simulink model "SecRwRtStHeightChk"  (R2018b)
settings: Solver=FixedStepDiscrete  StartTime=0.0  StopTime=10.0  FixedStep=0.01  RelTol=1e-3
undefined symbols (not defined in the file or in its folder): KeSMSeHeiCstTypeConfig_Val
libraries: simulink x3, HeightCalcLib x1
settings Model: Creator=sn2xws  LastModifiedBy=sn2xws
settings DataIOCC: SaveFormat=StructureWithTime
settings OptimizationCC: DefaultParameterBehavior=Inlined  EnhancedBackFolding=on  PassReuseOutputArgsAs=Individual arguments  ZeroExternalMemoryAtStartup=off  ZeroInternalMemoryAtStartup=off  OptimizeBlockOrder=speed  DifferentSizesBufferReuse=on  OptimizationCustomize=off
settings DebuggingCC: ParameterTunabilityLossMsg=error
settings ModelReferenceCC: ModelReferenceNumInstancesAllowed=Single
settings SFSimCC: MATLABDynamicMemAlloc=off
settings RTWCC: SystemTargetFile=autosar.tlc  GenCodeOnly=on  TemplateMakefile=ert_default_tmf  Description=AUTOSAR  GenerateReport=on  IncludeHyperlinkInReport=on  LaunchReport=on  GenerateTraceInfo=on  GenerateTraceReport=on  GenerateTraceReportSl=on  GenerateTraceReportSf=on  GenerateTraceReportEml=on  GenerateCodeMetricsReport=on
settings CodeAppCC: ForceParamTrailComments=on  IgnoreCustomStorageClasses=off  OperatorAnnotations=on  SimulinkDataObjDesc=on  SFDataObjDesc=on  InsertBlockDesc=on
settings STFCustomTargetCC: TargetLangStandard=C99 (ISO)  MultiwordLength=256  ParMdlRefBuildCompliant=on  CompOptLevelCompliant=on  IncludeMdlTerminateFcn=off  CombineOutputUpdateFcns=on  SuppressErrorStatus=on  ERTCustomFileBanners=on  SupportNonFinite=off  SupportComplex=off  SupportContinuousTime=off  SupportNonInlinedSFcns=off  RemoveResetFunc=on  MATLABClassNameForMDSCustomization=Simulink.SoftwareTarget.ERTCustomization  AutosarCompliant=on  UseToolchainInfoCompliant=on  LookupTableObjectStructAxisOrder=2,1,3,4,...  LUTObjectStructOrderEvenSpacing=Size,Table,Breakpoints  SystemTargetFile=autosar.tlc
settings ERTTargetCC: TargetLangStandard=C99 (ISO)  ConcurrentExecutionCompliant=off  IncludeMdlTerminateFcn=off  SuppressErrorStatus=on  SupportNonFinite=off  SupportComplex=off  ModelStepFunctionPrototypeControlCompliant=off  CPPClassGenCompliant=off  AutosarCompliant=on  LookupTableObjectStructAxisOrder=2,1,3,4,...  LUTObjectStructOrderEvenSpacing=Size,Table,Breakpoints  InlinedParameterPlacement=NonHierarchical  ERTCustomFileTemplate=example_file_process.tlc  ERTFilePackagingFormat=Compact

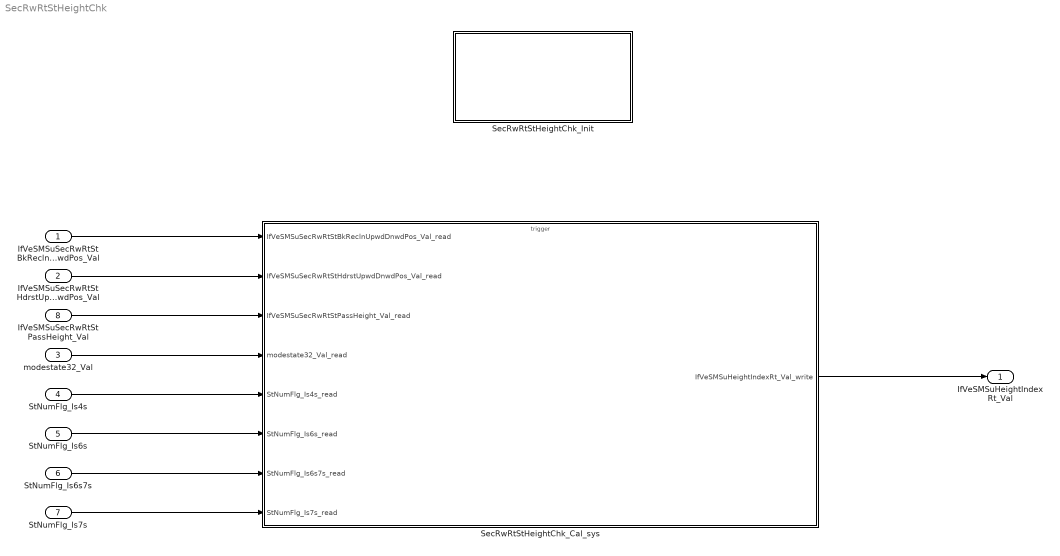
== system SecRwRtStHeightChk ==
  IfVeSMSuSecRwRtStBkReclnUpwdDnwdPos_Val : Inport  OutDataTypeStr=uint16  PortDimensions=1
  IfVeSMSuSecRwRtStHdrstUpwdDnwdPos_Val : Inport  Port=2  OutDataTypeStr=uint16  PortDimensions=1
  modestate32_Val : Inport  Port=3  OutDataTypeStr=uint32  PortDimensions=1
  StNumFlg_Is4s : Inport  Port=4  OutDataTypeStr=boolean  PortDimensions=1
  StNumFlg_Is6s : Inport  Port=5  OutDataTypeStr=boolean  PortDimensions=1
  StNumFlg_Is6s7s : Inport  Port=6  OutDataTypeStr=boolean  PortDimensions=1
  StNumFlg_Is7s : Inport  Port=7  OutDataTypeStr=boolean  PortDimensions=1
  IfVeSMSuSecRwRtStPassHeight_Val : Inport  Port=8  OutDataTypeStr=uint8  PortDimensions=1
  SecRwRtStHeightChk_Cal_sys : Subsystem
  SecRwRtStHeightChk_Init : Subsystem
  IfVeSMSuHeightIndexRt_Val : Outport  Description=|  OutDataTypeStr=uint8  PortDimensions=1
      | 0：under 160
      | 1：160
      | 2：165
      | 3：170
      | 4：175
      | 5：180
      | 6：over 180
  wires:
  IfVeSMSuSecRwRtStBkReclnUpwdDnwdPos_Val/1 -> SecRwRtStHeightChk_Cal_sys/1(IfVeSMSuSecRwRtStBkReclnUpwdDnwdPos_Val_read)
  IfVeSMSuSecRwRtStHdrstUpwdDnwdPos_Val/1 -> SecRwRtStHeightChk_Cal_sys/2(IfVeSMSuSecRwRtStHdrstUpwdDnwdPos_Val_read)
  modestate32_Val/1 -> SecRwRtStHeightChk_Cal_sys/4(modestate32_Val_read)
  StNumFlg_Is4s/1 -> SecRwRtStHeightChk_Cal_sys/5(StNumFlg_Is4s_read)
  StNumFlg_Is6s/1 -> SecRwRtStHeightChk_Cal_sys/6(StNumFlg_Is6s_read)
  StNumFlg_Is6s7s/1 -> SecRwRtStHeightChk_Cal_sys/7(StNumFlg_Is6s7s_read)
  StNumFlg_Is7s/1 -> SecRwRtStHeightChk_Cal_sys/8(StNumFlg_Is7s_read)
  IfVeSMSuSecRwRtStPassHeight_Val/1 -> SecRwRtStHeightChk_Cal_sys/3(IfVeSMSuSecRwRtStPassHeight_Val_read)
  SecRwRtStHeightChk_Cal_sys/1(IfVeSMSuHeightIndexRt_Val_write) -> IfVeSMSuHeightIndexRt_Val/1

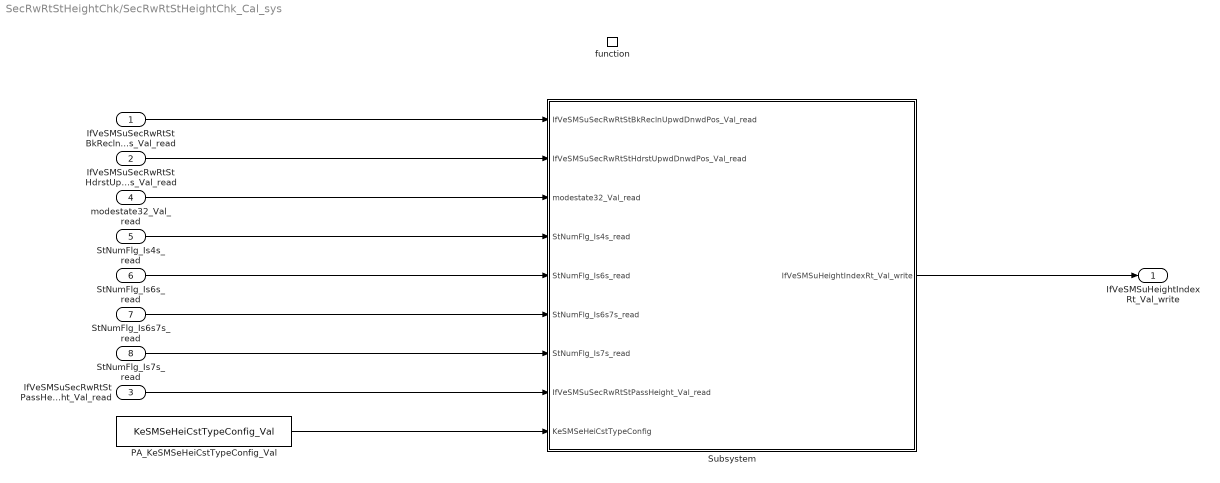
== system SecRwRtStHeightChk/SecRwRtStHeightChk_Cal_sys ==
  IfVeSMSuSecRwRtStBkReclnUpwdDnwdPos_Val_read : Inport
  IfVeSMSuSecRwRtStHdrstUpwdDnwdPos_Val_read : Inport  Port=2
  IfVeSMSuSecRwRtStPassHeight_Val_read : Inport  Port=3
  modestate32_Val_read : Inport  Port=4
  StNumFlg_Is4s_read : Inport  Port=5
  StNumFlg_Is6s_read : Inport  Port=6
  StNumFlg_Is6s7s_read : Inport  Port=7
  StNumFlg_Is7s_read : Inport  Port=8
  function : TriggerPort  TriggerType=function-call  IsSimulinkFunction=on  FunctionName=SecRwRtStHeightChk_Cal  VariantControl=(inherit)
  PA_KeSMSeHeiCstTypeConfig_Val : Constant  Value=KeSMSeHeiCstTypeConfig_Val
  Subsystem : Subsystem
  IfVeSMSuHeightIndexRt_Val_write : Outport
      settings: EnsureOutportIsVirtual=on
  wires:
  PA_KeSMSeHeiCstTypeConfig_Val/1 -> Subsystem/9(KeSMSeHeiCstTypeConfig)
  Subsystem/1(IfVeSMSuHeightIndexRt_Val_write) -> IfVeSMSuHeightIndexRt_Val_write/1
  IfVeSMSuSecRwRtStBkReclnUpwdDnwdPos_Val_read/1 -> Subsystem/1(IfVeSMSuSecRwRtStBkReclnUpwdDnwdPos_Val_read)
  IfVeSMSuSecRwRtStHdrstUpwdDnwdPos_Val_read/1 -> Subsystem/2(IfVeSMSuSecRwRtStHdrstUpwdDnwdPos_Val_read)
  modestate32_Val_read/1 -> Subsystem/3(modestate32_Val_read)
  StNumFlg_Is4s_read/1 -> Subsystem/4(StNumFlg_Is4s_read)
  StNumFlg_Is6s_read/1 -> Subsystem/5(StNumFlg_Is6s_read)
  StNumFlg_Is6s7s_read/1 -> Subsystem/6(StNumFlg_Is6s7s_read)
  StNumFlg_Is7s_read/1 -> Subsystem/7(StNumFlg_Is7s_read)
  IfVeSMSuSecRwRtStPassHeight_Val_read/1 -> Subsystem/8(IfVeSMSuSecRwRtStPassHeight_Val_read)

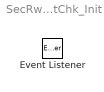
== system SecRwRtStHeightChk/SecRwRtStHeightChk_Init ==
  Event Listener : EventListener  EventName=reset

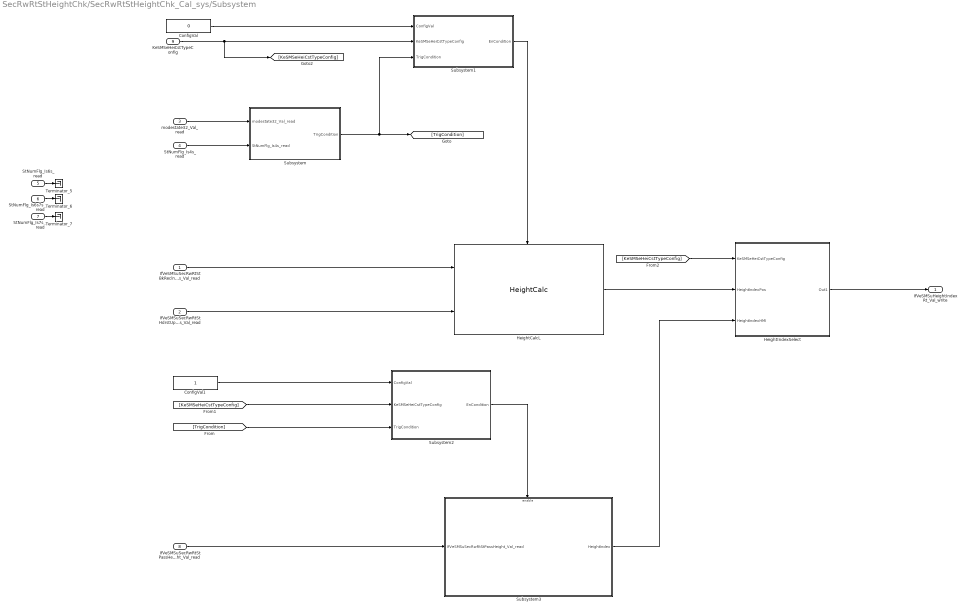
== system SecRwRtStHeightChk/SecRwRtStHeightChk_Cal_sys/Subsystem ==
  IfVeSMSuSecRwRtStBkReclnUpwdDnwdPos_Val_read : Inport
  IfVeSMSuSecRwRtStHdrstUpwdDnwdPos_Val_read : Inport  Port=2
  modestate32_Val_read : Inport  Port=3
  StNumFlg_Is4s_read : Inport  Port=4
  StNumFlg_Is6s_read : Inport  Port=5
  StNumFlg_Is6s7s_read : Inport  Port=6
  StNumFlg_Is7s_read : Inport  Port=7
  IfVeSMSuSecRwRtStPassHeight_Val_read : Inport  Port=8
  KeSMSeHeiCstTypeConfig : Inport  Port=9
  ConfigVal : Constant  Value=0  OutDataTypeStr=uint8
  ConfigVal1 : Constant  OutDataTypeStr=uint8
  HeightCalcL : HeightCalcLib/HeightCalc  SystemSampleTime=-1
  HeightIndexSelect : Subsystem
  Subsystem : Subsystem
  Subsystem1 : Subsystem
  Subsystem2 : Subsystem
  Subsystem3 : Subsystem
  Terminator_5 : Terminator
  Terminator_6 : Terminator
  Terminator_7 : Terminator
  IfVeSMSuHeightIndexRt_Val_write : Outport
      settings: EnsureOutportIsVirtual=on
  wires:
  IfVeSMSuSecRwRtStBkReclnUpwdDnwdPos_Val_read/1 -> HeightCalcL/1
  IfVeSMSuSecRwRtStHdrstUpwdDnwdPos_Val_read/1 -> HeightCalcL/2
  StNumFlg_Is6s_read/1 -> Terminator_5/1
  StNumFlg_Is7s_read/1 -> Terminator_7/1
  StNumFlg_Is6s7s_read/1 -> Terminator_6/1
  modestate32_Val_read/1 -> Subsystem/1(modestate32_Val_read)
  StNumFlg_Is4s_read/1 -> Subsystem/2(StNumFlg_Is4s_read)
  Subsystem1/1(EnCondition) -> HeightCalcL/Enable
  ConfigVal/1 -> Subsystem1/1(ConfigVal)
  ConfigVal1/1 -> Subsystem2/1(ConfigVal)
  KeSMSeHeiCstTypeConfig/1 -> [KeSMSeHeiCstTypeConfig], Subsystem1/2(KeSMSeHeiCstTypeConfig)
  [TrigCondition] -> Subsystem2/3(TrigCondition)
  [KeSMSeHeiCstTypeConfig] -> Subsystem2/2(KeSMSeHeiCstTypeConfig)
  IfVeSMSuSecRwRtStPassHeight_Val_read/1 -> Subsystem3/1(IfVeSMSuSecRwRtStPassHeight_Val_read)
  Subsystem2/1(EnCondition) -> Subsystem3/Enable
  HeightCalcL/1 -> HeightIndexSelect/2(HeightIndexPos)
  Subsystem3/1(HeightIndex) -> HeightIndexSelect/3(HeightIndexHMI)
  HeightIndexSelect/1(Out1) -> IfVeSMSuHeightIndexRt_Val_write/1
  [KeSMSeHeiCstTypeConfig] -> HeightIndexSelect/1(KeSMSeHeiCstTypeConfig)
  Subsystem/1(TrigCondition) -> [TrigCondition], Subsystem1/3(TrigCondition)

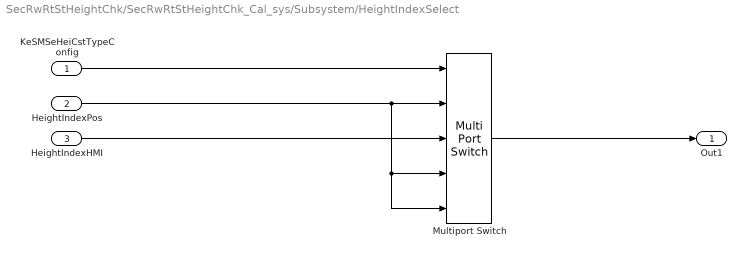
== system SecRwRtStHeightChk/SecRwRtStHeightChk_Cal_sys/Subsystem/HeightIndexSelect ==
  KeSMSeHeiCstTypeConfig : Inport
  HeightIndexPos : Inport  Port=2
  HeightIndexHMI : Inport  Port=3
  Multiport Switch : MultiPortSwitch  DataPortOrder=Zero-based contiguous  DataPortForDefault=Additional data port  DiagnosticForDefault=None  zeroidx=on
  Out1 : Outport
  wires:
  HeightIndexPos/1 -> Multiport Switch/5, Multiport Switch/4, Multiport Switch/2
  KeSMSeHeiCstTypeConfig/1 -> Multiport Switch/1
  Multiport Switch/1 -> Out1/1
  HeightIndexHMI/1 -> Multiport Switch/3

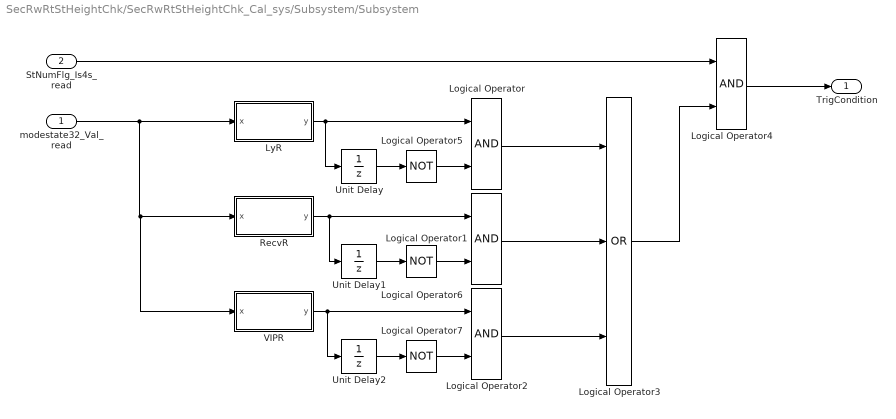
== system SecRwRtStHeightChk/SecRwRtStHeightChk_Cal_sys/Subsystem/Subsystem ==
  modestate32_Val_read : Inport
  StNumFlg_Is4s_read : Inport  Port=2
  Logical Operator{,1..2,4} (4 alike) : Logic  AllPortsSameDT=off  OutDataTypeStr=boolean
  Logical Operator3 : Logic  Operator=OR  Inputs=3  AllPortsSameDT=off  OutDataTypeStr=boolean
  Logical Operator5 : Logic  Operator=NOT  AllPortsSameDT=off  OutDataTypeStr=boolean
  Logical Operator6 : Logic  Operator=NOT  AllPortsSameDT=off  OutDataTypeStr=boolean
  Logical Operator7 : Logic  Operator=NOT  AllPortsSameDT=off  OutDataTypeStr=boolean
  LyR : Subsystem  mask(32 Bit Selector){BitNum=14}
      mask prompts: BitNum "Select Bit Number"
      mask help: Allows selection of a particular bit (0-31) out of a packed word up to 32 bits long. Output will be true if the bit number selected via the mask parameter is equal to one.
      mask TypeOptions BitNum: 0 | 1 | 2 | 3 | 4 | 5 | 6 | 7 | 8 | 9 | 10 | 11 | 12 | 13 | 14 | 15 | 16 | 17 | 18 | 19 | 20 | 21 | 22 | 23 | 24 | 25 | 26 | 27 | 28 | 29 | 30 | 31
      mask Display:
      | text(0.5, 0.8,'BIT','horizontalAlignment','center')
      | text(0.5, 0.5,'SELECTOR','horizontalAlignment','center')
      | text(0.5, 0.2,['-- Bit ',char(get_param(gcb,'BitNum')),' --'],'horizontalAlignment','center')
  RecvR : Subsystem  mask(32 Bit Selector){BitNum=12}
      mask prompts: BitNum "Select Bit Number"
      mask help: Allows selection of a particular bit (0-31) out of a packed word up to 32 bits long. Output will be true if the bit number selected via the mask parameter is equal to one.
      mask TypeOptions BitNum: 0 | 1 | 2 | 3 | 4 | 5 | 6 | 7 | 8 | 9 | 10 | 11 | 12 | 13 | 14 | 15 | 16 | 17 | 18 | 19 | 20 | 21 | 22 | 23 | 24 | 25 | 26 | 27 | 28 | 29 | 30 | 31
      mask Display:
      | text(0.5, 0.8,'BIT','horizontalAlignment','center')
      | text(0.5, 0.5,'SELECTOR','horizontalAlignment','center')
      | text(0.5, 0.2,['-- Bit ',char(get_param(gcb,'BitNum')),' --'],'horizontalAlignment','center')
  Unit Delay : UnitDelay  SampleTime=-1
  Unit Delay1 : UnitDelay  SampleTime=-1
  Unit Delay2 : UnitDelay  SampleTime=-1
  VIPR : Subsystem  mask(32 Bit Selector){BitNum=11}
      mask prompts: BitNum "Select Bit Number"
      mask help: Allows selection of a particular bit (0-31) out of a packed word up to 32 bits long. Output will be true if the bit number selected via the mask parameter is equal to one.
      mask TypeOptions BitNum: 0 | 1 | 2 | 3 | 4 | 5 | 6 | 7 | 8 | 9 | 10 | 11 | 12 | 13 | 14 | 15 | 16 | 17 | 18 | 19 | 20 | 21 | 22 | 23 | 24 | 25 | 26 | 27 | 28 | 29 | 30 | 31
      mask Display:
      | text(0.5, 0.8,'BIT','horizontalAlignment','center')
      | text(0.5, 0.5,'SELECTOR','horizontalAlignment','center')
      | text(0.5, 0.2,['-- Bit ',char(get_param(gcb,'BitNum')),' --'],'horizontalAlignment','center')
  TrigCondition : Outport
  wires:
  VIPR/1(y) -> Unit Delay2/1, Logical Operator2/1
  RecvR/1(y) -> Unit Delay1/1, Logical Operator1/1
  StNumFlg_Is4s_read/1 -> Logical Operator4/1
  LyR/1(y) -> Unit Delay/1, Logical Operator/1
  Logical Operator2/1 -> Logical Operator3/3
  modestate32_Val_read/1 -> VIPR/1(x), RecvR/1(x), LyR/1(x)
  Logical Operator3/1 -> Logical Operator4/2
  Logical Operator1/1 -> Logical Operator3/2
  Logical Operator/1 -> Logical Operator3/1
  Logical Operator4/1 -> TrigCondition/1
  Unit Delay/1 -> Logical Operator5/1
  Logical Operator5/1 -> Logical Operator/2
  Unit Delay1/1 -> Logical Operator6/1
  Logical Operator6/1 -> Logical Operator1/2
  Unit Delay2/1 -> Logical Operator7/1
  Logical Operator7/1 -> Logical Operator2/2

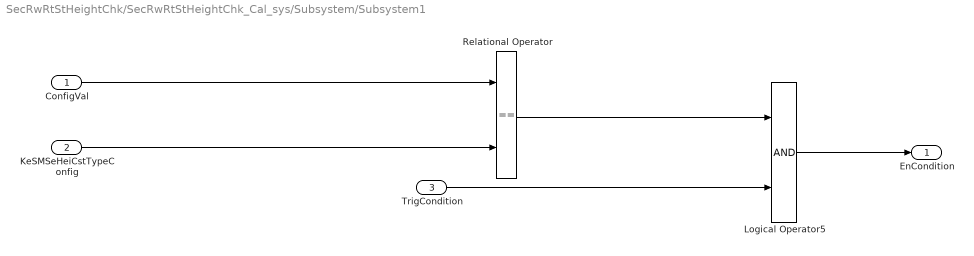
== system SecRwRtStHeightChk/SecRwRtStHeightChk_Cal_sys/Subsystem/Subsystem1 ==
  ConfigVal : Inport
  KeSMSeHeiCstTypeConfig : Inport  Port=2
  TrigCondition : Inport  Port=3
  Logical Operator5 : Logic  AllPortsSameDT=off  OutDataTypeStr=boolean
  Relational Operator : RelationalOperator  Operator===  OutDataTypeStr=boolean  RndMeth=Simplest
  EnCondition : Outport
  wires:
  Logical Operator5/1 -> EnCondition/1
  Relational Operator/1 -> Logical Operator5/1
  KeSMSeHeiCstTypeConfig/1 -> Relational Operator/2
  ConfigVal/1 -> Relational Operator/1
  TrigCondition/1 -> Logical Operator5/2

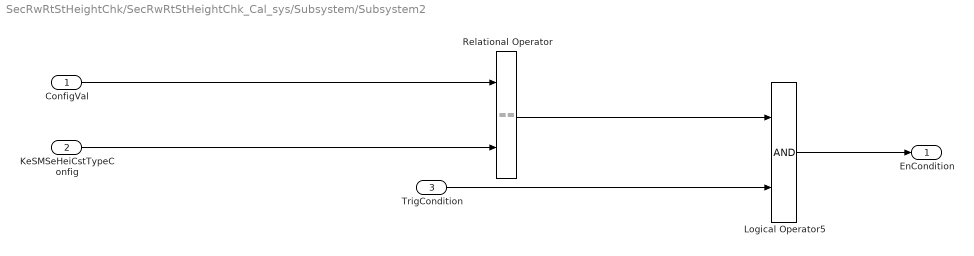
== system SecRwRtStHeightChk/SecRwRtStHeightChk_Cal_sys/Subsystem/Subsystem2 ==
  ConfigVal : Inport
  KeSMSeHeiCstTypeConfig : Inport  Port=2
  TrigCondition : Inport  Port=3
  Logical Operator5 : Logic  AllPortsSameDT=off  OutDataTypeStr=boolean
  Relational Operator : RelationalOperator  Operator===  OutDataTypeStr=boolean  RndMeth=Simplest
  EnCondition : Outport
  wires:
  TrigCondition/1 -> Logical Operator5/2
  ConfigVal/1 -> Relational Operator/1
  KeSMSeHeiCstTypeConfig/1 -> Relational Operator/2
  Relational Operator/1 -> Logical Operator5/1
  Logical Operator5/1 -> EnCondition/1

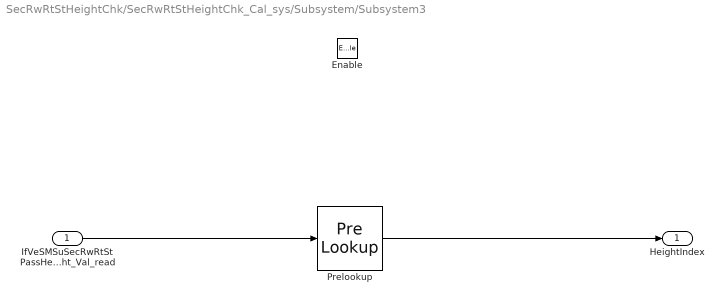
== system SecRwRtStHeightChk/SecRwRtStHeightChk_Cal_sys/Subsystem/Subsystem3 ==
  IfVeSMSuSecRwRtStPassHeight_Val_read : Inport
  Enable : EnablePort
  Prelookup : PreLookup  BreakpointsData=HeightIndexR  OutputSelection=Index only  RemoveProtectionInput=on  IndexDataTypeStr=uint8
  HeightIndex : Outport
  wires:
  Prelookup/1 -> HeightIndex/1
  IfVeSMSuSecRwRtStPassHeight_Val_read/1 -> Prelookup/1

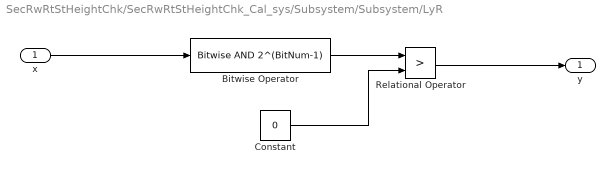
== system SecRwRtStHeightChk/SecRwRtStHeightChk_Cal_sys/Subsystem/Subsystem/LyR ==
  x : Inport
  Bitwise Operator : simulink/Logic and Bit Operations/Bitwise Operator  logicop=AND  UseBitMask=on  BitMask=2^(BitNum-1)  BitMaskRealWorld=Stored Integer
  Constant : Constant  Value=0  OutDataTypeStr=uint32
  Relational Operator : RelationalOperator  Operator=>  OutDataTypeStr=boolean  RndMeth=Simplest
  y : Outport
  wires:
  Relational Operator/1 -> y/1
  Constant/1 -> Relational Operator/2
  x/1 -> Bitwise Operator/1
  Bitwise Operator/1 -> Relational Operator/1

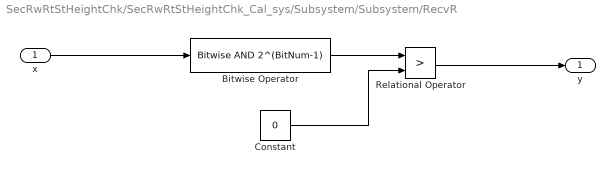
== system SecRwRtStHeightChk/SecRwRtStHeightChk_Cal_sys/Subsystem/Subsystem/RecvR ==
  x : Inport
  Bitwise Operator : simulink/Logic and Bit Operations/Bitwise Operator  logicop=AND  UseBitMask=on  BitMask=2^(BitNum-1)  BitMaskRealWorld=Stored Integer
  Constant : Constant  Value=0  OutDataTypeStr=uint32
  Relational Operator : RelationalOperator  Operator=>  OutDataTypeStr=boolean  RndMeth=Simplest
  y : Outport
  wires:
  Bitwise Operator/1 -> Relational Operator/1
  x/1 -> Bitwise Operator/1
  Constant/1 -> Relational Operator/2
  Relational Operator/1 -> y/1

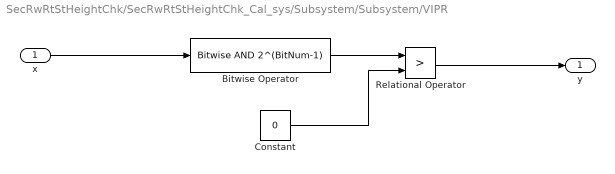
== system SecRwRtStHeightChk/SecRwRtStHeightChk_Cal_sys/Subsystem/Subsystem/VIPR ==
  x : Inport
  Bitwise Operator : simulink/Logic and Bit Operations/Bitwise Operator  logicop=AND  UseBitMask=on  BitMask=2^(BitNum-1)  BitMaskRealWorld=Stored Integer
  Constant : Constant  Value=0  OutDataTypeStr=uint32
  Relational Operator : RelationalOperator  Operator=>  OutDataTypeStr=boolean  RndMeth=Simplest
  y : Outport
  wires:
  Relational Operator/1 -> y/1
  Constant/1 -> Relational Operator/2
  x/1 -> Bitwise Operator/1
  Bitwise Operator/1 -> Relational Operator/1
